simulink model "DCMLab5"  (R2021a)
settings: Solver=VariableStepAuto  StartTime=0.0  StopTime=10.0  RelTol=1e-3
settings Model: Creator=manram  LastModifiedBy=manram

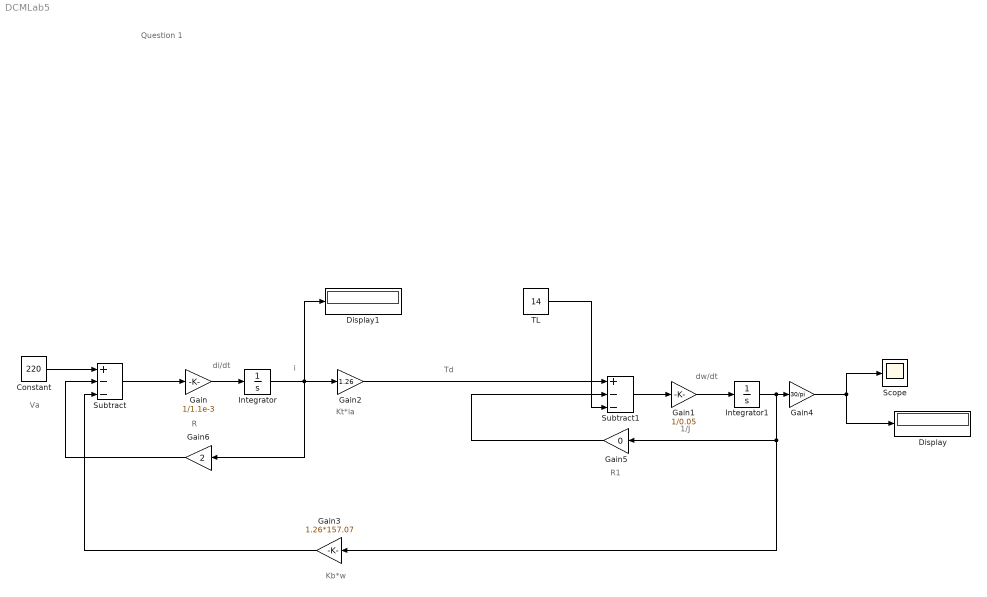
== system DCMLab5 ==
  note: Question 1
  note: Td
  note: dw/dt
  note: 1/J
  note: Kb*w
  note: Kt*ia
  note: R1
  note: di/dt
  note: i
  note: R
  note: Va
  Constant : Constant  Value=220
  Display : Display
  Display1 : Display
  Gain : Gain  Gain=1/1.1e-3
  Gain1 : Gain  Gain=1/0.05
  Gain2 : Gain  Gain=1.26
  Gain3 : Gain  Gain=1.26*157.07
  Gain4 : Gain  Gain=30/pi
  Gain5 : Gain  Gain=0
  Gain6 : Gain  Gain=2
  Integrator : Integrator
  Integrator1 : Integrator
  Scope : Scope
  Subtract : Sum  Inputs=+--
  Subtract1 : Sum  Inputs=+--
  TL : Constant  Value=14
  wires:
  Subtract/1 -> Gain/1
  Constant/1 -> Subtract/1
  Subtract1/1 -> Gain1/1
  TL/1 -> Subtract1/3
  Gain2/1 -> Subtract1/1
  Gain3/1 -> Subtract/3
  Gain4/1 -> Display/1, Scope/1
  Gain5/1 -> Subtract1/2
  Gain/1 -> Integrator/1
  Integrator/1 -> Display1/1, Gain6/1, Gain2/1
  Gain1/1 -> Integrator1/1
  Integrator1/1 -> Gain3/1, Gain5/1, Gain4/1
  Gain6/1 -> Subtract/2
